simulink model "Tra_RtnIntfc"  (R2016b)
settings: configuration reference "CodeGenConfigSet" (kept outside this file)
values from neighbouring files (symbols this model uses):
  Tra_bCANIdlSetP_C = Calibration.Parameter    [init_Tra_RtnIntfc.m]
  Tra_bFltIdlSpdDes_C = Calibration.Parameter    [init_Tra_RtnIntfc.m]
  Tra_nMax_C = Calibration.Parameter    [init_Tra_RtnIntfc.m]
  Tra_nMin_C = Calibration.Parameter    [init_Tra_RtnIntfc.m]
  TRA_STNSETP_FLT = fi(0,State_uint8)    [init_Tra_RtnIntfc.m]
  TRA_STNSETP_UNFLT = fi(1,State_uint8)    [init_Tra_RtnIntfc.m]
settings Model: Creator=Colin  LastModifiedBy=Colin
settings ConfigSetRef: SourceLocation=Base Workspace

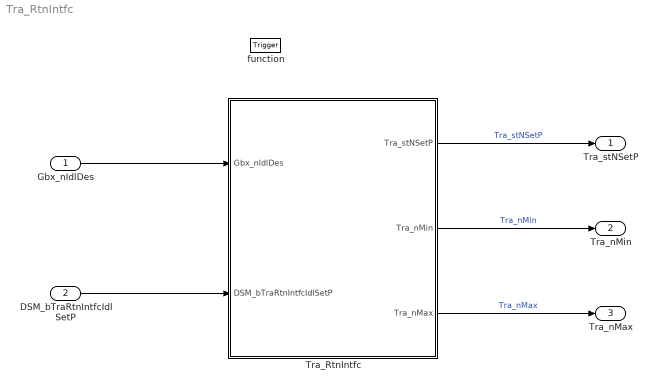
== system Tra_RtnIntfc ==
  Gbx_nIdlDes : Inport  Tag=rpm  Description=Desired idle speed setpoint for AT gear box rpm  OutMin=-6000  OutMax=6000  OutDataTypeStr=EngSpeed_rpm
  DSM_bTraRtnIntfcIdlSetP : Inport  Description=Fault Indicator low-idle setpoint speed increase via CAN  Port=2  OutMin=0  OutMax=1  OutDataTypeStr=boolean
  function : TriggerPort  TriggerType=function-call  VariantControl=Variant
  Tra_RtnIntfc : Subsystem
  Tra_stNSetP : Outport  Description=Status for current set point engine speed requirement  OutMin=0  OutMax=255  OutDataTypeStr=State_uint8
  Tra_nMin : Outport  Tag=rpm  Description=Minimum engine speed for gearbox  Port=2  OutMin=-6000  OutMax=6000  OutDataTypeStr=EngSpeed_rpm
  Tra_nMax : Outport  Tag=rpm  Description=Maximum engine speed for gearbox  Port=3  OutMin=-6000  OutMax=11000  OutDataTypeStr=EngSpeed_rpm
  wires:
  Tra_RtnIntfc/1(Tra_stNSetP) -> Tra_stNSetP/1  "Tra_stNSetP"
  Tra_RtnIntfc/2(Tra_nMin) -> Tra_nMin/1  "Tra_nMin"
  Tra_RtnIntfc/3(Tra_nMax) -> Tra_nMax/1  "Tra_nMax"
  Gbx_nIdlDes/1 -> Tra_RtnIntfc/1(Gbx_nIdlDes)
  DSM_bTraRtnIntfcIdlSetP/1 -> Tra_RtnIntfc/2(DSM_bTraRtnIntfcIdlSetP)

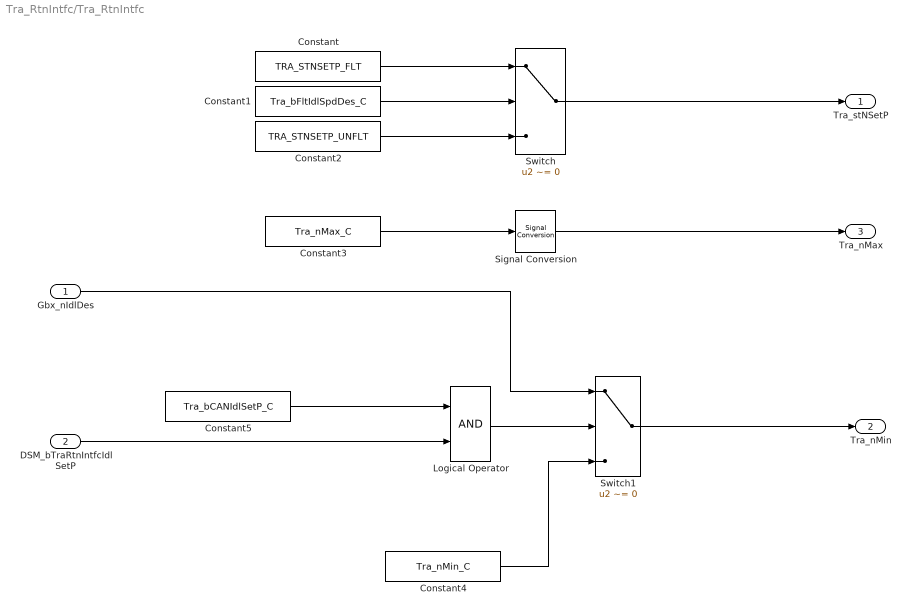
== system Tra_RtnIntfc/Tra_RtnIntfc ==
  Gbx_nIdlDes : Inport  Tag=rpm  Description=Desired idle speed setpoint for AT gear box rpm  OutMin=-6000  OutMax=6000  OutDataTypeStr=EngSpeed_rpm
  DSM_bTraRtnIntfcIdlSetP : Inport  Port=2
  Constant : Constant  Value=TRA_STNSETP_FLT
  Constant1 : Constant  Value=Tra_bFltIdlSpdDes_C
  Constant2 : Constant  Value=TRA_STNSETP_UNFLT
  Constant3 : Constant  Value=Tra_nMax_C
  Constant4 : Constant  Value=Tra_nMin_C
  Constant5 : Constant  Value=Tra_bCANIdlSetP_C
  Logical Operator : Logic  AllPortsSameDT=off  OutDataTypeStr=boolean
  Signal Conversion : SignalConversion  OverrideOpt=off
  Switch : Switch  Criteria=u2 ~= 0
  Switch1 : Switch  Criteria=u2 ~= 0
  Tra_stNSetP : Outport  Description=Status for current set point engine speed requirement  OutMin=0  OutMax=255  OutDataTypeStr=State_uint8
  Tra_nMin : Outport  Tag=rpm  Description=Minimum engine speed for gearbox  Port=2  OutMin=-6000  OutMax=6000  OutDataTypeStr=EngSpeed_rpm
  Tra_nMax : Outport  Tag=rpm  Description=Maximum engine speed for gearbox  Port=3  OutMin=-6000  OutMax=11000  OutDataTypeStr=EngSpeed_rpm
  wires:
  Switch/1 -> Tra_stNSetP/1
  Switch1/1 -> Tra_nMin/1
  Signal Conversion/1 -> Tra_nMax/1
  Constant5/1 -> Logical Operator/1
  Logical Operator/1 -> Switch1/2
  Constant4/1 -> Switch1/3
  Gbx_nIdlDes/1 -> Switch1/1
  DSM_bTraRtnIntfcIdlSetP/1 -> Logical Operator/2
  Constant3/1 -> Signal Conversion/1
  Constant/1 -> Switch/1
  Constant1/1 -> Switch/2
  Constant2/1 -> Switch/3
